simulink model "Simulink_Crippa_DiMauro"  (R2024b)
settings: Solver=VariableStepAuto  StartTime=0.0  StopTime=50  RelTol=1e-3
values from neighbouring files (symbols this model uses):
  B1 = 0.05    [MatlabCode_Crippa_DiMauro.m]
  Beq = 0.015    [MatlabCode_Crippa_DiMauro.m]
  bias_opampl = 1.65    [MatlabCode_Crippa_DiMauro.m]
  eta_g = 0.90    (= 0.9)    [MatlabCode_Crippa_DiMauro.m]
  eta_m = 0.85    [MatlabCode_Crippa_DiMauro.m]
  J1 = 0.025    [MatlabCode_Crippa_DiMauro.m]
  Jeq = 0.0022    [MatlabCode_Crippa_DiMauro.m]
  K1 = 1.5    [MatlabCode_Crippa_DiMauro.m]
  K_opampl = 2.75    [MatlabCode_Crippa_DiMauro.m]
  K_transducerVel = (10e-3)/(pi/180)    (= 0.572957795131)    [MatlabCode_Crippa_DiMauro.m]
  kd_vel = (zero1_vel*zero2_vel)*ki_vel-kp_vel*pole1_vel    (= 0.026)    [MatlabCode_Crippa_DiMauro.m]
  Kg = 70    [MatlabCode_Crippa_DiMauro.m]
  ki_vel = gain_vel    (= 20)    [MatlabCode_Crippa_DiMauro.m]
  Km = 7.68e-3    (= 0.00768)    [MatlabCode_Crippa_DiMauro.m]
  kp_vel = (zero1_vel+zero2_vel)*ki_vel-ki_vel*pole1_vel    (= 3.2)    [MatlabCode_Crippa_DiMauro.m]
  Kpo = wcouter/mu_q    [MatlabCode_Crippa_DiMauro.m]
  Kt = 7.68e-3    (= 0.00768)    [MatlabCode_Crippa_DiMauro.m]
  N_choose11 = 11    [MatlabCode_Crippa_DiMauro.m]
  N_choose9 = 9    [MatlabCode_Crippa_DiMauro.m]
  Ra = 10    [MatlabCode_Crippa_DiMauro.m]
  tau_f = 0.02    [MatlabCode_Crippa_DiMauro.m]
  TdelayADCPos = 11e-6    (= 1.1e-05)    [MatlabCode_Crippa_DiMauro.m]
  TdelayADCVel = 9e-6    (= 9e-06)    [MatlabCode_Crippa_DiMauro.m]
  Ts = 0.02    [MatlabCode_Crippa_DiMauro.m]
  Vfs = 3.3    [MatlabCode_Crippa_DiMauro.m]
libraries: dspfdesign x2, slpidlib x2
settings Model: Creator=matti  LastModifiedBy=matti
settings ConfigComp: CovBoundaryAbsTol=1.0e-5

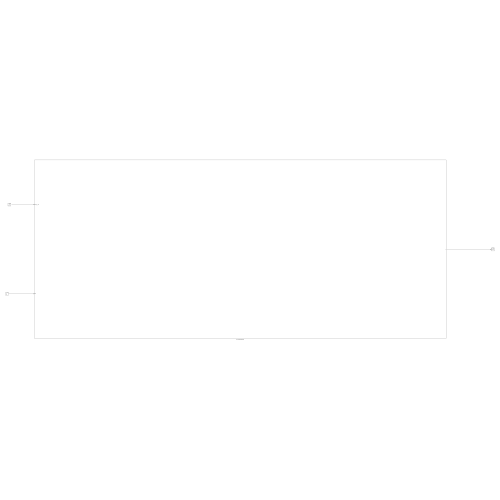
[thumbnail: Simulink's stored preview of the top-level diagram]
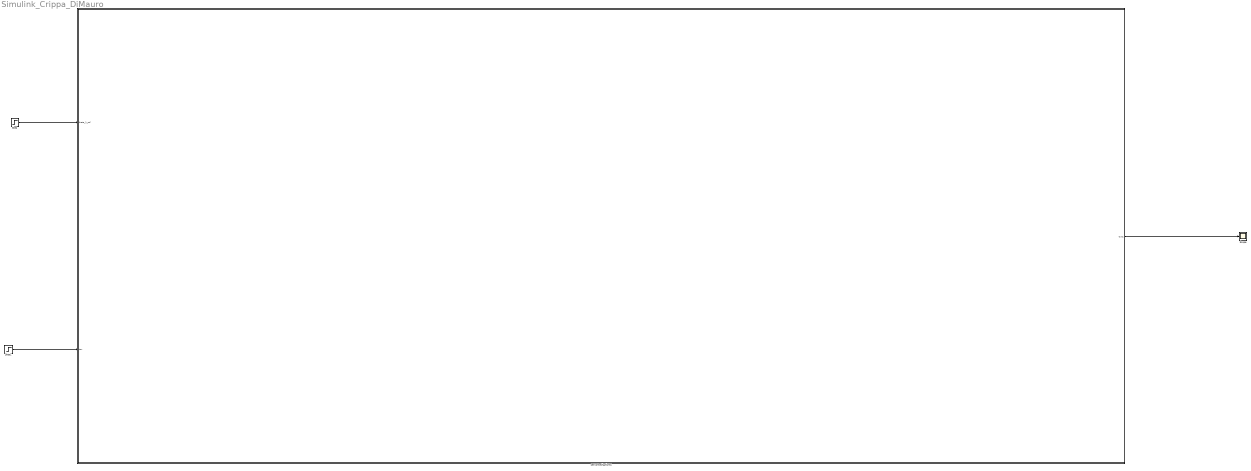
== system Simulink_Crippa_DiMauro ==
  Scope : Scope
  Step : Step  Time=0  After=30*pi/180  SampleTime=0
  Step1 : Step  Time=5  After=0.5  SampleTime=0
  servomechanisms : Subsystem
  wires:
  Step1/1 -> servomechanisms/2(tau)
  servomechanisms/1(Out1) -> Scope/1
  Step/1 -> servomechanisms/1(theta_1_ref)

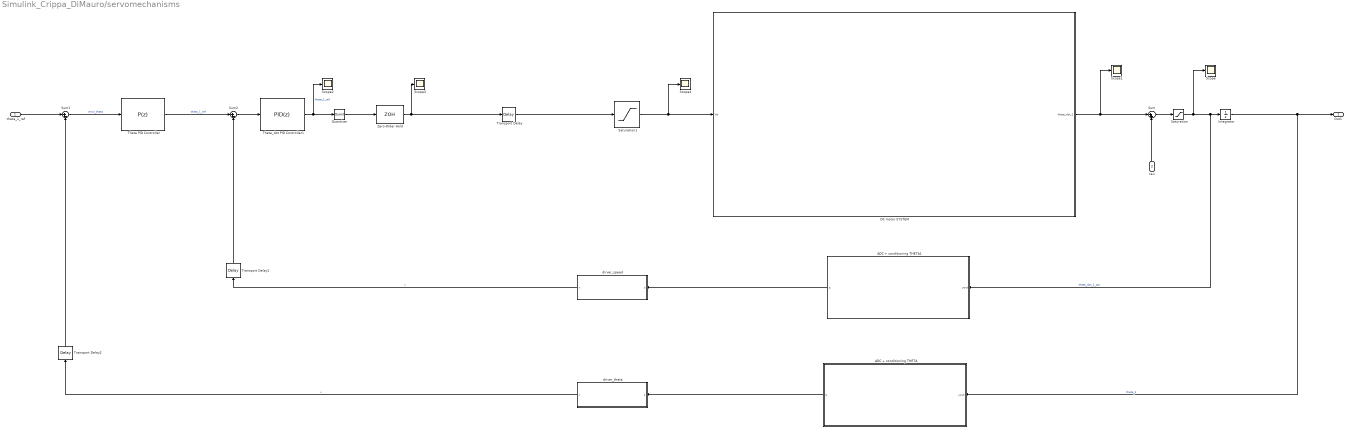
== system Simulink_Crippa_DiMauro/servomechanisms ==
  theta_1_ref : Inport
  tau : Inport  Port=2
  ADC + conditioning THETA : Subsystem
  ADC + conditioning THETA1 : Subsystem
  DC motor SYSTEM : Subsystem
  Integrator : Integrator
  Quantizer : Quantizer  QuantizationInterval=LSB_quantizer
  Saturation : Saturate  UpperLimit=45*pi/180  LowerLimit=-45*pi/180
  Saturation1 : Saturate  UpperLimit=12  LowerLimit=-12
  Scope{,1..4} (5 alike) : Scope
  Sum : Sum  Inputs=|++
  Sum1 : Sum  Inputs=|+-
  Sum2 : Sum  Inputs=|+-
  Theta PID Controller : slpidlib/PID Controller  Controller=P  Form=Parallel  TimeDomain=Discrete-time  UseExternalTs=off  SampleTime=Ts  IntegratorMethod=Forward Euler  FilterMethod=Forward Euler  ControllerParametersSource=internal  P=Kpo  I=1  UseKiTs=off  D=0  UseExternalDerivativeSource=off  N=100  UseFilter=on  TunerSelectOption=Transfer Function Based (PID Tuner App)  InitialConditionSource=internal  InitialConditionForIntegrator=0  InitialConditionForFilter=0  DifferentiatorICPrevScaledInput=0  ExternalReset=none  TrackingMode=off  Kt=1  LimitOutput=off  SatLimitsSource=internal  UpperSaturationLimit=inf  LowerSaturationLimit=-inf  LinearizeAsGain=on  AntiWindupMode=none  Kb=1  LimitIntegrator=off  UpperIntegratorSaturationLimit=inf  LowerIntegratorSaturationLimit=-inf  POutMin=[]  POutMax=[]  IOutMin=[]  IOutMax=[]  DOutMin=[]  DOutMax=[]  NOutMin=[]  NOutMax=[]  SumOutMin=[]  SumOutMax=[]  SaturationOutMin=[]  SaturationOutMax=[]  PParamMin=[]  PParamMax=[]  IParamMin=[]  IParamMax=[]  DParamMin=[]  DParamMax=[]  NParamMin=[]  NParamMax=[]  KbParamMin=[]  KbParamMax=[]  KtParamMin=[]  KtParamMax=[]  KbOutMin=[]  KbOutMax=[]  KtOutMin=[]  KtOutMax=[]  IntegratorOutMin=[]  IntegratorOutMax=[]  FilterOutMin=[]  FilterOutMax=[]  SumI1OutMin=[]  SumI1OutMax=[]  SumI2OutMin=[]  SumI2OutMax=[]  SumI3OutMin=[]  SumI3OutMax=[]  SumI4OutMin=[]  SumI4OutMax=[]  SumDOutMin=[]  SumDOutMax=[]  DifferentiatorOutMin=[]  DifferentiatorOutMax=[]  FilterDiffOutCoefMin=[]  FilterDiffOutCoefMax=[]  ReciprocalOutMin=[]  ReciprocalOutMax=[]  SumDenOutMin=[]  SumDenOutMax=[]  SumNumOutMin=[]  SumNumOutMax=[]  DivideOutMin=[]  DivideOutMax=[]  UdiffTsProdOutMin=[]  UdiffTsProdOutMax=[]  NTsProdOutMin=[]  NTsProdOutMax=[]  UintegralTsProdOutMin=[]  UintegralTsProdOutMax=[]  UngainTsProdOutMin=[]  UngainTsProdOutMax=[]  ClampingZeroOutDataTypeStr=Inherit: Inherit via back propagation  ClampingZeroOutMin=[]  ClampingZeroOutMax=[]  FilterDenConstantOutDataTypeStr=Inherit: Inherit via back propagation  FilterDenConstantOutMin=[]  FilterDenConstantOutMax=[]  PCopyOutDataTypeStr=Inherit: Inherit via back propagation  PCopyOutMin=[]  PCopyOutMax=[]  NCopyOutDataTypeStr=Inherit: Inherit via back propagation  NCopyOutMin=[]  NCopyOutMax=[]  IntegratorContinuousStateAttributes=''  IntegratorStateMustResolveToSignalObject=off  IntegratorRTWStateStorageClass=Auto  FilterContinuousStateAttributes=''  FilterStateMustResolveToSignalObject=off  FilterRTWStateStorageClass=Auto  ParallelPVariant=InternalParameters  IdealPVariant=Disabled  IVariant=Disabled  DVariant=Disabled  IntegratorVariant=Disabled  SatVariant=Disabled  AWVariant=Disabled  PCopyVariant=Disabled  TRVariant=Disabled  FdbkBlocksVariant=Forward  IdealPFdbkVariant=Disabled  SatFdbkVariant=Disabled  DerivativeFilterVariant=Disabled  NVariant=Disabled  NCopyVariant=Disabled_SignalSpec  FilterICVariant=Disabled  IntegratorICVariant=Disabled  ExternalResetVariant=Disabled  TRSumVariant=Passthrough  SumFdbkVariant=Disabled  SumVariant=Passthrough_P  TsampFilterVariant=InternalTs  TsampNgainVariant=Passthrough  TsampIntegralVariant=Disabled_SignalSpec  ExternalSaturationOutDataTypeStr=Inherit: Same as second input  DerivativeSourceVariant=Disabled  PreIntVariant=InternalPreInt
  Theta_dot PID Controller1 : slpidlib/PID Controller  Controller=PID  Form=Parallel  TimeDomain=Discrete-time  UseExternalTs=off  SampleTime=Ts  IntegratorMethod=Forward Euler  FilterMethod=Forward Euler  ControllerParametersSource=internal  P=kp_vel  I=ki_vel  UseKiTs=off  D=kd_vel  UseExternalDerivativeSource=off  N=1/tau_f  UseFilter=on  TunerSelectOption=Transfer Function Based (PID Tuner App)  InitialConditionSource=internal  InitialConditionForIntegrator=0  InitialConditionForFilter=0  DifferentiatorICPrevScaledInput=0  ExternalReset=none  TrackingMode=off  Kt=1  LimitOutput=on  SatLimitsSource=internal  UpperSaturationLimit=inf  LowerSaturationLimit=-inf  LinearizeAsGain=on  AntiWindupMode=back-calculation  Kb=1  LimitIntegrator=off  UpperIntegratorSaturationLimit=inf  LowerIntegratorSaturationLimit=-inf  POutMin=[]  POutMax=[]  IOutMin=[]  IOutMax=[]  DOutMin=[]  DOutMax=[]  NOutMin=[]  NOutMax=[]  SumOutMin=[]  SumOutMax=[]  SaturationOutMin=[]  SaturationOutMax=[]  PParamMin=[]  PParamMax=[]  IParamMin=[]  IParamMax=[]  DParamMin=[]  DParamMax=[]  NParamMin=[]  NParamMax=[]  KbParamMin=[]  KbParamMax=[]  KtParamMin=[]  KtParamMax=[]  KbOutMin=[]  KbOutMax=[]  KtOutMin=[]  KtOutMax=[]  IntegratorOutMin=[]  IntegratorOutMax=[]  FilterOutMin=[]  FilterOutMax=[]  SumI1OutMin=[]  SumI1OutMax=[]  SumI2OutMin=[]  SumI2OutMax=[]  SumI3OutMin=[]  SumI3OutMax=[]  SumI4OutMin=[]  SumI4OutMax=[]  SumDOutMin=[]  SumDOutMax=[]  DifferentiatorOutMin=[]  DifferentiatorOutMax=[]  FilterDiffOutCoefMin=[]  FilterDiffOutCoefMax=[]  ReciprocalOutMin=[]  ReciprocalOutMax=[]  SumDenOutMin=[]  SumDenOutMax=[]  SumNumOutMin=[]  SumNumOutMax=[]  DivideOutMin=[]  DivideOutMax=[]  UdiffTsProdOutMin=[]  UdiffTsProdOutMax=[]  NTsProdOutMin=[]  NTsProdOutMax=[]  UintegralTsProdOutMin=[]  UintegralTsProdOutMax=[]  UngainTsProdOutMin=[]  UngainTsProdOutMax=[]  ClampingZeroOutDataTypeStr=Inherit: Inherit via back propagation  ClampingZeroOutMin=[]  ClampingZeroOutMax=[]  FilterDenConstantOutDataTypeStr=Inherit: Inherit via back propagation  FilterDenConstantOutMin=[]  FilterDenConstantOutMax=[]  PCopyOutDataTypeStr=Inherit: Inherit via back propagation  PCopyOutMin=[]  PCopyOutMax=[]  NCopyOutDataTypeStr=Inherit: Inherit via back propagation  NCopyOutMin=[]  NCopyOutMax=[]  IntegratorContinuousStateAttributes=''  IntegratorStateMustResolveToSignalObject=off  IntegratorRTWStateStorageClass=Auto  FilterContinuousStateAttributes=''  FilterStateMustResolveToSignalObject=off  FilterRTWStateStorageClass=Auto  ParallelPVariant=InternalParameters  IdealPVariant=Disabled  IVariant=InternalParameters  DVariant=InternalParameters  IntegratorVariant=Discrete  SatVariant=Enabled  AWVariant=BackCalculation  PCopyVariant=Disabled  TRVariant=Disabled  FdbkBlocksVariant=Forward  IdealPFdbkVariant=Disabled  SatFdbkVariant=Disabled  DerivativeFilterVariant=ForwardEulerFilter  NVariant=InternalParameters  NCopyVariant=Disabled  FilterICVariant=InternalICsFilter  IntegratorICVariant=InternalICs  ExternalResetVariant=Disabled  TRSumVariant=Passthrough  SumFdbkVariant=Disabled  SumVariant=Sum_PID  TsampFilterVariant=InternalTs  TsampNgainVariant=Passthrough  TsampIntegralVariant=Disabled_SignalSpec  ExternalSaturationOutDataTypeStr=Inherit: Same as second input  DerivativeSourceVariant=ErrorSignal  PreIntVariant=InternalPreInt
  Transport Delay : TransportDelay  DelayTime=Ts/2
  Transport Delay1 : TransportDelay  DelayTime=TdelayADCVel
  Transport Delay2 : TransportDelay  DelayTime=TdelayADCPos
  Zero-Order Hold : ZeroOrderHold  SampleTime=Ts
  dirver_speed : Subsystem
  driver_theta : Subsystem
  Out1 : Outport
  wires:
  tau/1 -> Sum/2
  theta_1_ref/1 -> Sum1/1
  Saturation/1 -> Scope/1, Integrator/1, ADC + conditioning THETA1/1(yout)  "theta_dot_1_sat"
  Saturation1/1 -> Scope4/1, DC motor SYSTEM/1(Va)
  Integrator/1 -> Out1/1, ADC + conditioning THETA/1(yout)  "theta_1"
  Sum2/1 -> Theta_dot PID Controller1/1
  Sum1/1 -> Theta PID Controller/1  "error_theta"
  DC motor SYSTEM/1(theta_dot_1) -> Scope1/1, Sum/1
  Theta PID Controller/1 -> Sum2/1  "theta_1_ref"
  Sum/1 -> Saturation/1
  ADC + conditioning THETA/1(q) -> driver_theta/1(s)
  ADC + conditioning THETA1/1(q) -> dirver_speed/1(s)
  Quantizer/1 -> Zero-Order Hold/1
  Zero-Order Hold/1 -> Transport Delay/1, Scope3/1
  Theta_dot PID Controller1/1 -> Quantizer/1, Scope2/1  "theta_1_ref"
  Transport Delay/1 -> Saturation1/1
  driver_theta/1(v) -> Transport Delay2/1  "v"
  Transport Delay2/1 -> Sum1/2
  Transport Delay1/1 -> Sum2/2
  dirver_speed/1(v) -> Transport Delay1/1  "v"

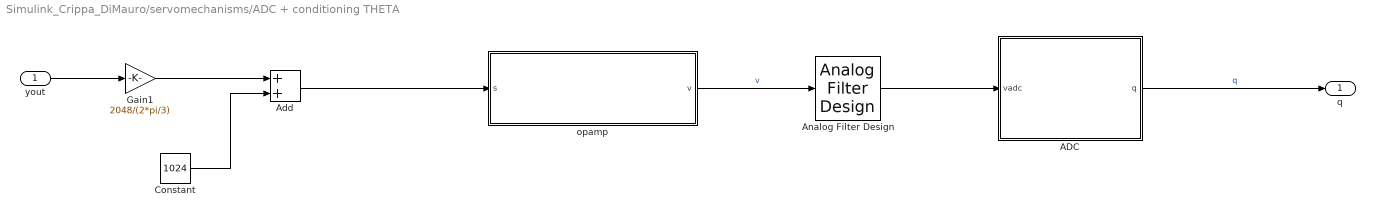
== system Simulink_Crippa_DiMauro/servomechanisms/ADC + conditioning THETA ==
  yout : Inport
  ADC : Subsystem
  Add : Sum
  Analog Filter Design : dspfdesign/Analog Filter Design  method=Butterworth  filttype=Lowpass  N=2  Wlo=w_AA  Whi=80  Rp=2  Rs=40
  Constant : Constant  Value=1024
  Gain1 : Gain  Gain=2048/(2*pi/3)
  opamp : Subsystem
  q : Outport
  wires:
  ADC/1(q) -> q/1  "q"
  yout/1 -> Gain1/1
  Gain1/1 -> Add/1
  Constant/1 -> Add/2
  Add/1 -> opamp/1(s)
  Analog Filter Design/1 -> ADC/1(vadc)
  opamp/1(v) -> Analog Filter Design/1  "v"

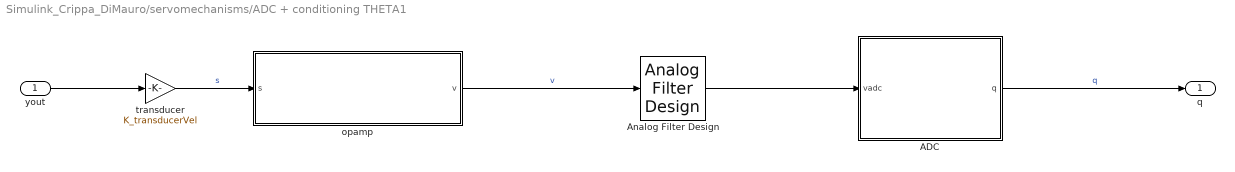
== system Simulink_Crippa_DiMauro/servomechanisms/ADC + conditioning THETA1 ==
  yout : Inport
  ADC : Subsystem
  Analog Filter Design : dspfdesign/Analog Filter Design  method=Butterworth  filttype=Lowpass  N=2  Wlo=w_AA  Whi=80  Rp=2  Rs=40
  opamp : Subsystem
  transducer : Gain  Gain=K_transducerVel
  q : Outport
  wires:
  yout/1 -> transducer/1
  transducer/1 -> opamp/1(s)  "s"
  ADC/1(q) -> q/1  "q"
  Analog Filter Design/1 -> ADC/1(vadc)
  opamp/1(v) -> Analog Filter Design/1  "v"

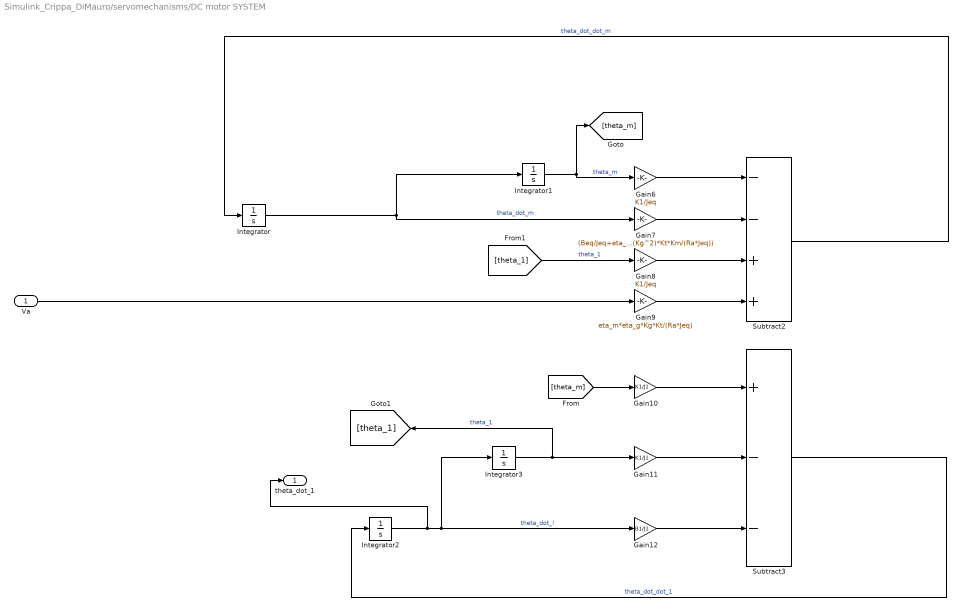
== system Simulink_Crippa_DiMauro/servomechanisms/DC motor SYSTEM ==
  Va : Inport
  Gain10 : Gain  Gain=K1/J1
  Gain11 : Gain  Gain=K1/J1
  Gain12 : Gain  Gain=B1/J1
  Gain6 : Gain  Gain=K1/Jeq
  Gain7 : Gain  Gain=(Beq/Jeq+eta_m*eta_g*(Kg^2)*Kt*Km/(Ra*Jeq))
  Gain8 : Gain  Gain=K1/Jeq
  Gain9 : Gain  Gain=eta_m*eta_g*Kg*Kt/(Ra*Jeq)
  Integrator{,1..3} (4 alike) : Integrator
  Subtract2 : Sum  Inputs=--++
  Subtract3 : Sum  Inputs=+--
  theta_dot_1 : Outport
  wires:
  Subtract3/1 -> Integrator2/1  "theta_dot_dot_1"
  [theta_m] -> Gain10/1
  Gain7/1 -> Subtract2/2
  Gain9/1 -> Subtract2/4
  Gain12/1 -> Subtract3/3
  Gain6/1 -> Subtract2/1
  Integrator3/1 -> [theta_1], Gain11/1  "theta_1"
  Integrator/1 -> Integrator1/1, Gain7/1  "theta_dot_m"
  Integrator1/1 -> Gain6/1, [theta_m]  "theta_m"
  Subtract2/1 -> Integrator/1  "theta_dot_dot_m"
  Gain8/1 -> Subtract2/3
  Va/1 -> Gain9/1
  Gain10/1 -> Subtract3/1
  Integrator2/1 -> theta_dot_1/1, Integrator3/1, Gain12/1  "theta_dot_!"
  [theta_1] -> Gain8/1  "theta_1"
  Gain11/1 -> Subtract3/2

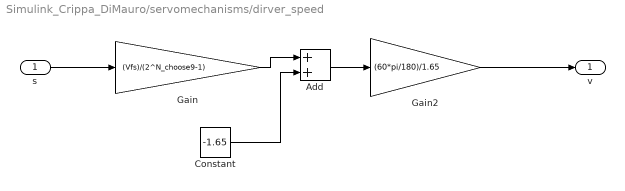
== system Simulink_Crippa_DiMauro/servomechanisms/dirver_speed ==
  s : Inport
  Add : Sum
  Constant : Constant  Value=-1.65
  Gain : Gain  Gain=(Vfs)/(2^N_choose9-1)
  Gain2 : Gain  Gain=(60*pi/180)/1.65
  v : Outport
  wires:
  s/1 -> Gain/1
  Add/1 -> Gain2/1
  Gain/1 -> Add/1
  Constant/1 -> Add/2
  Gain2/1 -> v/1

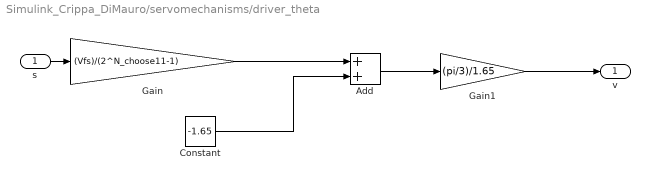
== system Simulink_Crippa_DiMauro/servomechanisms/driver_theta ==
  s : Inport
  Add : Sum
  Constant : Constant  Value=-1.65
  Gain : Gain  Gain=(Vfs)/(2^N_choose11-1)
  Gain1 : Gain  Gain=(pi/3)/1.65
  v : Outport
  wires:
  s/1 -> Gain/1
  Add/1 -> Gain1/1
  Gain1/1 -> v/1
  Gain/1 -> Add/1
  Constant/1 -> Add/2

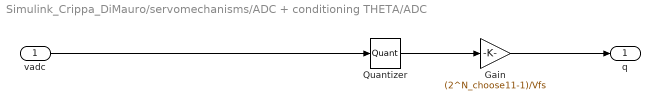
== system Simulink_Crippa_DiMauro/servomechanisms/ADC + conditioning THETA/ADC ==
  vadc : Inport
  Gain : Gain  Gain=(2^N_choose11-1)/Vfs
  Quantizer : Quantizer  QuantizationInterval=LSB_11
  q : Outport
  wires:
  Gain/1 -> q/1
  Quantizer/1 -> Gain/1
  vadc/1 -> Quantizer/1

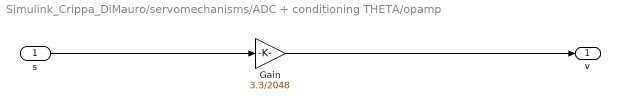
== system Simulink_Crippa_DiMauro/servomechanisms/ADC + conditioning THETA/opamp ==
  s : Inport
  Gain : Gain  Gain=3.3/2048
  v : Outport
  wires:
  s/1 -> Gain/1
  Gain/1 -> v/1

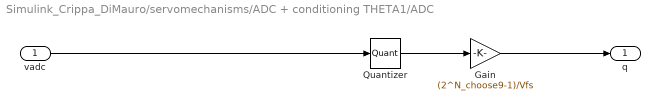
== system Simulink_Crippa_DiMauro/servomechanisms/ADC + conditioning THETA1/ADC ==
  vadc : Inport
  Gain : Gain  Gain=(2^N_choose9-1)/Vfs
  Quantizer : Quantizer  QuantizationInterval=LSB_9
  q : Outport
  wires:
  vadc/1 -> Quantizer/1
  Quantizer/1 -> Gain/1
  Gain/1 -> q/1

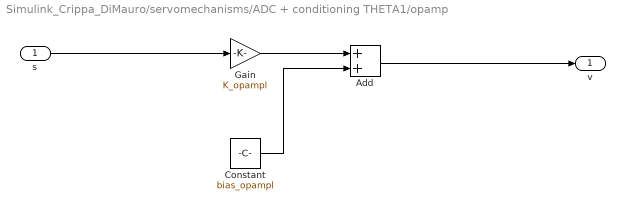
== system Simulink_Crippa_DiMauro/servomechanisms/ADC + conditioning THETA1/opamp ==
  s : Inport
  Add : Sum
  Constant : Constant  Value=bias_opampl
  Gain : Gain  Gain=K_opampl
  v : Outport
  wires:
  Add/1 -> v/1
  s/1 -> Gain/1
  Gain/1 -> Add/1
  Constant/1 -> Add/2
